simulink model "vsi_fmt_core"  (Simulink 7.0)
settings: Solver=ode45  StartTime=0.0  StopTime=10.0  RelTol=1e-3
libraries: xbsIndex_r4 x293, xbsReplacements_r4 x15, simulink x3, vlbi_lib x1
(part 2 of 2)

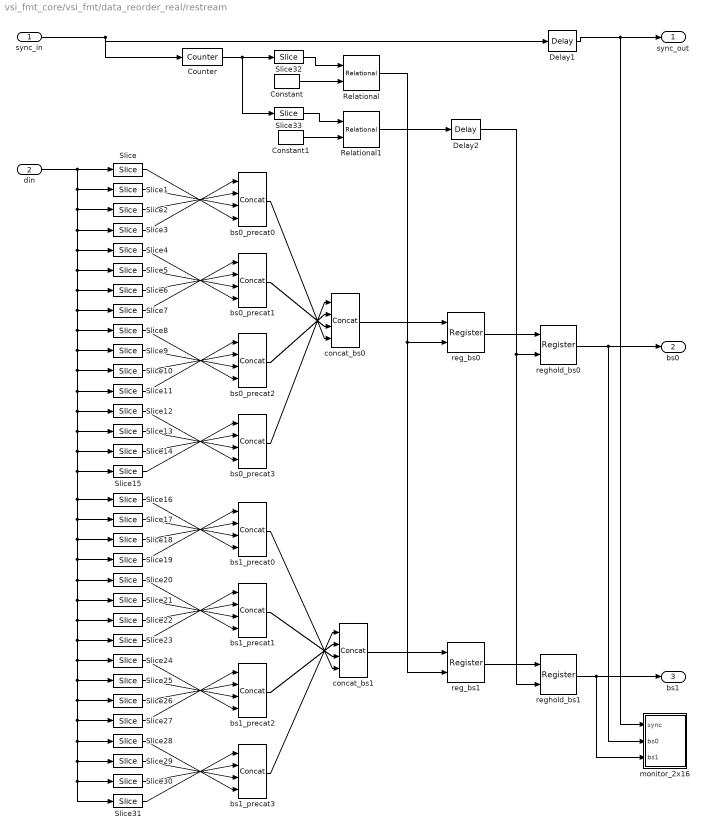
== system vsi_fmt_core/vsi_fmt/data_reorder_real/restream ==
  sync_in : Inport  OutDataType=sfix(16)  OutScaling=2^0
  din : Inport  Port=2  OutDataType=sfix(16)  OutScaling=2^0
  Constant : xbsIndex_r4/Constant  arith_type=Unsigned  const=0  n_bits=8-log2(clock_rate)  bin_pt=0  explicit_period=on  period=1  equ=P=C  opselect=C  inp2=PCIN>>17  opr=+  inp1=P  carry=CIN  dbl_ovrd=off  block_type=constant
      settings: block_version=11.3
  Constant1 : xbsIndex_r4/Constant  arith_type=Unsigned  const=0  n_bits=8-log2(clock_rate)  bin_pt=0  explicit_period=on  period=1  equ=P=C  opselect=C  inp2=PCIN>>17  opr=+  inp1=P  carry=CIN  dbl_ovrd=off  block_type=constant
      settings: block_version=11.3
  Counter : xbsIndex_r4/Counter  cnt_type=Free Running  cnt_to=Inf  operation=Up  start_count=0  cnt_by_val=1  arith_type=Unsigned  n_bits=9-log2(clock_rate)  bin_pt=0  load_pin=off  rst=on  en=off  explicit_period=off  period=1  dbl_ovrd=off  use_behavioral_HDL=off  use_rpm=on  implementation=Fabric  block_type=counter
      settings: xl_area=[0, 0, 0, 0, 0, 0, 0]  block_version=11.3
  Delay1 : xbsIndex_r4/Delay  en=off  latency=2  dbl_ovrd=off  reg_retiming=off  block_type=delay
      settings: xl_area=[0, 0, 0, 0, 0, 0, 0]  block_version=11.3
  Delay2 : xbsIndex_r4/Delay  en=off  latency=1  dbl_ovrd=off  reg_retiming=off  block_type=delay
      settings: xl_area=[0, 0, 0, 0, 0, 0, 0]  block_version=11.3
  Relational : xbsIndex_r4/Relational  mode=a=b  en=off  latency=0  dbl_ovrd=off  block_type=relational
      settings: xl_area=[0, 0, 0, 0, 0, 0, 0]  block_version=11.3
  Relational1 : xbsIndex_r4/Relational  mode=a=b  en=off  latency=0  dbl_ovrd=off  block_type=relational
      settings: xl_area=[0, 0, 0, 0, 0, 0, 0]  block_version=11.3
  Slice : xbsIndex_r4/Slice  nbits=sample_width  boolean_output=off  mode=Lower Bit Location + Width  bit1=sample_width*0  base1=MSB of Input  bit0=sample_width*7  base0=LSB of Input  dbl_ovrd=off  block_type=slice
      settings: block_version=11.3
  Slice1 : xbsIndex_r4/Slice  nbits=sample_width  boolean_output=off  mode=Lower Bit Location + Width  bit1=-2*sample_width  base1=MSB of Input  bit0=sample_width*6  base0=LSB of Input  dbl_ovrd=off  block_type=slice
      settings: block_version=11.3
  Slice10 : xbsIndex_r4/Slice  nbits=sample_width  boolean_output=off  mode=Lower Bit Location + Width  bit1=sample_width*21  base1=MSB of Input  bit0=sample_width*21  base0=LSB of Input  dbl_ovrd=off  block_type=slice
      settings: block_version=11.3
  Slice11 : xbsIndex_r4/Slice  nbits=sample_width  boolean_output=off  mode=Lower Bit Location + Width  bit1=-22*sample_width  base1=MSB of Input  bit0=sample_width*20  base0=LSB of Input  dbl_ovrd=off  block_type=slice
      settings: block_version=11.3
  Slice12 : xbsIndex_r4/Slice  nbits=sample_width  boolean_output=off  mode=Lower Bit Location + Width  bit1=-24*sample_width  base1=MSB of Input  bit0=sample_width*31  base0=LSB of Input  dbl_ovrd=off  block_type=slice
      settings: block_version=11.3
  Slice13 : xbsIndex_r4/Slice  nbits=sample_width  boolean_output=off  mode=Lower Bit Location + Width  bit1=-26*sample_width  base1=MSB of Input  bit0=sample_width*30  base0=LSB of Input  dbl_ovrd=off  block_type=slice
      settings: block_version=11.3
  Slice14 : xbsIndex_r4/Slice  nbits=sample_width  boolean_output=off  mode=Lower Bit Location + Width  bit1=-28*sample_width  base1=MSB of Input  bit0=sample_width*29  base0=LSB of Input  dbl_ovrd=off  block_type=slice
      settings: block_version=11.3
  Slice15 : xbsIndex_r4/Slice  nbits=sample_width  boolean_output=off  mode=Lower Bit Location + Width  bit1=-30*sample_width  base1=MSB of Input  bit0=sample_width*28  base0=LSB of Input  dbl_ovrd=off  block_type=slice
      settings: block_version=11.3
  Slice16 : xbsIndex_r4/Slice  nbits=sample_width  boolean_output=off  mode=Lower Bit Location + Width  bit1=-1*sample_width  base1=MSB of Input  bit0=sample_width*3  base0=LSB of Input  dbl_ovrd=off  block_type=slice
      settings: block_version=11.3
  Slice17 : xbsIndex_r4/Slice  nbits=sample_width  boolean_output=off  mode=Lower Bit Location + Width  bit1=-3*sample_width  base1=MSB of Input  bit0=sample_width*2  base0=LSB of Input  dbl_ovrd=off  block_type=slice
      settings: block_version=11.3
  Slice18 : xbsIndex_r4/Slice  nbits=sample_width  boolean_output=off  mode=Lower Bit Location + Width  bit1=-5*sample_width  base1=MSB of Input  bit0=sample_width*1  base0=LSB of Input  dbl_ovrd=off  block_type=slice
      settings: block_version=11.3
  Slice19 : xbsIndex_r4/Slice  nbits=sample_width  boolean_output=off  mode=Lower Bit Location + Width  bit1=-7*sample_width  base1=MSB of Input  bit0=sample_width*0  base0=LSB of Input  dbl_ovrd=off  block_type=slice
      settings: block_version=11.3
  Slice2 : xbsIndex_r4/Slice  nbits=sample_width  boolean_output=off  mode=Lower Bit Location + Width  bit1=-4*sample_width  base1=MSB of Input  bit0=sample_width*5  base0=LSB of Input  dbl_ovrd=off  block_type=slice
      settings: block_version=11.3
  Slice20 : xbsIndex_r4/Slice  nbits=sample_width  boolean_output=off  mode=Lower Bit Location + Width  bit1=-9*sample_width  base1=MSB of Input  bit0=sample_width*11  base0=LSB of Input  dbl_ovrd=off  block_type=slice
      settings: block_version=11.3
  Slice21 : xbsIndex_r4/Slice  nbits=sample_width  boolean_output=off  mode=Lower Bit Location + Width  bit1=-11*sample_width  base1=MSB of Input  bit0=sample_width*10  base0=LSB of Input  dbl_ovrd=off  block_type=slice
      settings: block_version=11.3
  Slice22 : xbsIndex_r4/Slice  nbits=sample_width  boolean_output=off  mode=Lower Bit Location + Width  bit1=-13*sample_width  base1=MSB of Input  bit0=sample_width*9  base0=LSB of Input  dbl_ovrd=off  block_type=slice
      settings: block_version=11.3
  Slice23 : xbsIndex_r4/Slice  nbits=sample_width  boolean_output=off  mode=Lower Bit Location + Width  bit1=-15*sample_width  base1=MSB of Input  bit0=sample_width*8  base0=LSB of Input  dbl_ovrd=off  block_type=slice
      settings: block_version=11.3
  Slice24 : xbsIndex_r4/Slice  nbits=sample_width  boolean_output=off  mode=Lower Bit Location + Width  bit1=-17*sample_width  base1=MSB of Input  bit0=sample_width*19  base0=LSB of Input  dbl_ovrd=off  block_type=slice
      settings: block_version=11.3
  Slice25 : xbsIndex_r4/Slice  nbits=sample_width  boolean_output=off  mode=Lower Bit Location + Width  bit1=sample_width*18  base1=MSB of Input  bit0=sample_width*18  base0=LSB of Input  dbl_ovrd=off  block_type=slice
      settings: block_version=11.3
  Slice26 : xbsIndex_r4/Slice  nbits=sample_width  boolean_output=off  mode=Lower Bit Location + Width  bit1=-21*sample_width  base1=MSB of Input  bit0=sample_width*17  base0=LSB of Input  dbl_ovrd=off  block_type=slice
      settings: block_version=11.3
  Slice27 : xbsIndex_r4/Slice  nbits=sample_width  boolean_output=off  mode=Lower Bit Location + Width  bit1=-23*sample_width  base1=MSB of Input  bit0=sample_width*16  base0=LSB of Input  dbl_ovrd=off  block_type=slice
      settings: block_version=11.3
  Slice28 : xbsIndex_r4/Slice  nbits=sample_width  boolean_output=off  mode=Lower Bit Location + Width  bit1=-25*sample_width  base1=MSB of Input  bit0=sample_width*27  base0=LSB of Input  dbl_ovrd=off  block_type=slice
      settings: block_version=11.3
  Slice29 : xbsIndex_r4/Slice  nbits=sample_width  boolean_output=off  mode=Lower Bit Location + Width  bit1=-27*sample_width  base1=MSB of Input  bit0=sample_width*26  base0=LSB of Input  dbl_ovrd=off  block_type=slice
      settings: block_version=11.3
  Slice3 : xbsIndex_r4/Slice  nbits=sample_width  boolean_output=off  mode=Lower Bit Location + Width  bit1=-6*sample_width  base1=MSB of Input  bit0=sample_width*4  base0=LSB of Input  dbl_ovrd=off  block_type=slice
      settings: block_version=11.3
  Slice30 : xbsIndex_r4/Slice  nbits=sample_width  boolean_output=off  mode=Lower Bit Location + Width  bit1=-29*sample_width  base1=MSB of Input  bit0=sample_width*25  base0=LSB of Input  dbl_ovrd=off  block_type=slice
      settings: block_version=11.3
  Slice31 : xbsIndex_r4/Slice  nbits=sample_width  boolean_output=off  mode=Lower Bit Location + Width  bit1=-31*sample_width  base1=MSB of Input  bit0=sample_width*24  base0=LSB of Input  dbl_ovrd=off  block_type=slice
      settings: block_version=11.3
  Slice32 : xbsIndex_r4/Slice  nbits=8-log2(clock_rate)  boolean_output=off  mode=Upper Bit Location + Width  bit1=0  base1=MSB of Input  bit0=sample_width*7  base0=LSB of Input  dbl_ovrd=off  block_type=slice
      settings: block_version=11.3
  Slice33 : xbsIndex_r4/Slice  nbits=8-log2(clock_rate)  boolean_output=off  mode=Lower Bit Location + Width  bit1=0  base1=MSB of Input  bit0=0  base0=LSB of Input  dbl_ovrd=off  block_type=slice
      settings: block_version=11.3
  Slice4 : xbsIndex_r4/Slice  nbits=sample_width  boolean_output=off  mode=Lower Bit Location + Width  bit1=-8*sample_width  base1=MSB of Input  bit0=sample_width*15  base0=LSB of Input  dbl_ovrd=off  block_type=slice
      settings: block_version=11.3
  Slice5 : xbsIndex_r4/Slice  nbits=sample_width  boolean_output=off  mode=Lower Bit Location + Width  bit1=-10*sample_width  base1=MSB of Input  bit0=sample_width*14  base0=LSB of Input  dbl_ovrd=off  block_type=slice
      settings: block_version=11.3
  Slice6 : xbsIndex_r4/Slice  nbits=sample_width  boolean_output=off  mode=Lower Bit Location + Width  bit1=-12*sample_width  base1=MSB of Input  bit0=sample_width*13  base0=LSB of Input  dbl_ovrd=off  block_type=slice
      settings: block_version=11.3
  Slice7 : xbsIndex_r4/Slice  nbits=sample_width  boolean_output=off  mode=Lower Bit Location + Width  bit1=-14*sample_width  base1=MSB of Input  bit0=sample_width*12  base0=LSB of Input  dbl_ovrd=off  block_type=slice
      settings: block_version=11.3
  Slice8 : xbsIndex_r4/Slice  nbits=sample_width  boolean_output=off  mode=Lower Bit Location + Width  bit1=-16*sample_width  base1=MSB of Input  bit0=sample_width*23  base0=LSB of Input  dbl_ovrd=off  block_type=slice
      settings: block_version=11.3
  Slice9 : xbsIndex_r4/Slice  nbits=sample_width  boolean_output=off  mode=Lower Bit Location + Width  bit1=-18*sample_width  base1=MSB of Input  bit0=sample_width*22  base0=LSB of Input  dbl_ovrd=off  block_type=slice
      settings: block_version=11.3
  bs0_precat{0..3} (4 alike) : xbsIndex_r4/Concat  num_inputs=4  dbl_ovrd=off  block_type=concat
      settings: block_version=11.3
  bs1_precat{0..3} (4 alike) : xbsIndex_r4/Concat  num_inputs=4  dbl_ovrd=off  block_type=concat
      settings: block_version=11.3
  concat_bs0 : xbsIndex_r4/Concat  num_inputs=4  dbl_ovrd=off  block_type=concat
      settings: block_version=11.3
  concat_bs1 : xbsIndex_r4/Concat  num_inputs=4  dbl_ovrd=off  block_type=concat
      settings: block_version=11.3
  monitor_2x16 : Subsystem
  reg_bs0 : xbsIndex_r4/Register  init=0  rst=off  en=on  dbl_ovrd=off  block_type=register
      settings: xl_area=[0, 0, 0, 0, 0, 0, 0]  block_version=11.3
  reg_bs1 : xbsIndex_r4/Register  init=0  rst=off  en=on  dbl_ovrd=off  block_type=register
      settings: xl_area=[0, 0, 0, 0, 0, 0, 0]  block_version=11.3
  reghold_bs0 : xbsIndex_r4/Register  init=0  rst=off  en=on  dbl_ovrd=off  block_type=register
      settings: xl_area=[0, 0, 0, 0, 0, 0, 0]  block_version=11.3
  reghold_bs1 : xbsIndex_r4/Register  init=0  rst=off  en=on  dbl_ovrd=off  block_type=register
      settings: xl_area=[0, 0, 0, 0, 0, 0, 0]  block_version=11.3
  sync_out : Outport  OutDataType=sfix(16)  OutScaling=2^0
  bs0 : Outport  Port=2  OutDataType=sfix(16)  OutScaling=2^0
  bs1 : Outport  Port=3  OutDataType=sfix(16)  OutScaling=2^0
  wires:
  Delay2/1 -> reghold_bs1/2, reghold_bs0/2
  Relational1/1 -> Delay2/1
  Slice33/1 -> Relational1/1
  Constant1/1 -> Relational1/2
  Slice32/1 -> Relational/1
  Counter/1 -> Slice33/1, Slice32/1
  reghold_bs1/1 -> monitor_2x16/3(bs1), bs1/1
  reghold_bs0/1 -> monitor_2x16/2(bs0), bs0/1
  Delay1/1 -> monitor_2x16/1(sync), sync_out/1
  reg_bs1/1 -> reghold_bs1/1
  reg_bs0/1 -> reghold_bs0/1
  Relational/1 -> reg_bs1/2, reg_bs0/2
  Constant/1 -> Relational/2
  sync_in/1 -> Delay1/1, Counter/1
  din/1 -> Slice6/1, Slice7/1, Slice14/1, Slice15/1, Slice16/1, Slice17/1, Slice18/1, Slice19/1, Slice20/1, Slice21/1, Slice24/1, Slice25/1, Slice26/1, Slice27/1, Slice28/1, Slice29/1, Slice30/1, Slice31/1, Slice23/1, Slice22/1, Slice13/1, Slice12/1, Slice11/1, Slice10/1, Slice9/1, Slice8/1, Slice5/1, Slice4/1, Slice3/1, Slice2/1, Slice1/1, Slice/1
  Slice/1 -> bs0_precat0/4
  Slice1/1 -> bs0_precat0/3
  Slice2/1 -> bs0_precat0/2
  Slice3/1 -> bs0_precat0/1
  Slice4/1 -> bs0_precat1/4
  Slice5/1 -> bs0_precat1/3
  Slice6/1 -> bs0_precat1/2
  Slice7/1 -> bs0_precat1/1
  Slice8/1 -> bs0_precat2/4
  Slice9/1 -> bs0_precat2/3
  Slice10/1 -> bs0_precat2/2
  Slice11/1 -> bs0_precat2/1
  Slice12/1 -> bs0_precat3/4
  Slice13/1 -> bs0_precat3/3
  Slice14/1 -> bs0_precat3/2
  Slice15/1 -> bs0_precat3/1
  Slice16/1 -> bs1_precat0/4
  Slice17/1 -> bs1_precat0/3
  Slice18/1 -> bs1_precat0/2
  Slice19/1 -> bs1_precat0/1
  Slice20/1 -> bs1_precat1/4
  Slice21/1 -> bs1_precat1/3
  Slice22/1 -> bs1_precat1/2
  Slice23/1 -> bs1_precat1/1
  Slice24/1 -> bs1_precat2/4
  Slice25/1 -> bs1_precat2/3
  Slice26/1 -> bs1_precat2/2
  Slice27/1 -> bs1_precat2/1
  Slice28/1 -> bs1_precat3/4
  Slice29/1 -> bs1_precat3/3
  Slice30/1 -> bs1_precat3/2
  Slice31/1 -> bs1_precat3/1
  concat_bs0/1 -> reg_bs0/1
  concat_bs1/1 -> reg_bs1/1
  bs0_precat0/1 -> concat_bs0/4
  bs0_precat1/1 -> concat_bs0/3
  bs0_precat2/1 -> concat_bs0/2
  bs0_precat3/1 -> concat_bs0/1
  bs1_precat0/1 -> concat_bs1/4
  bs1_precat1/1 -> concat_bs1/3
  bs1_precat2/1 -> concat_bs1/2
  bs1_precat3/1 -> concat_bs1/1

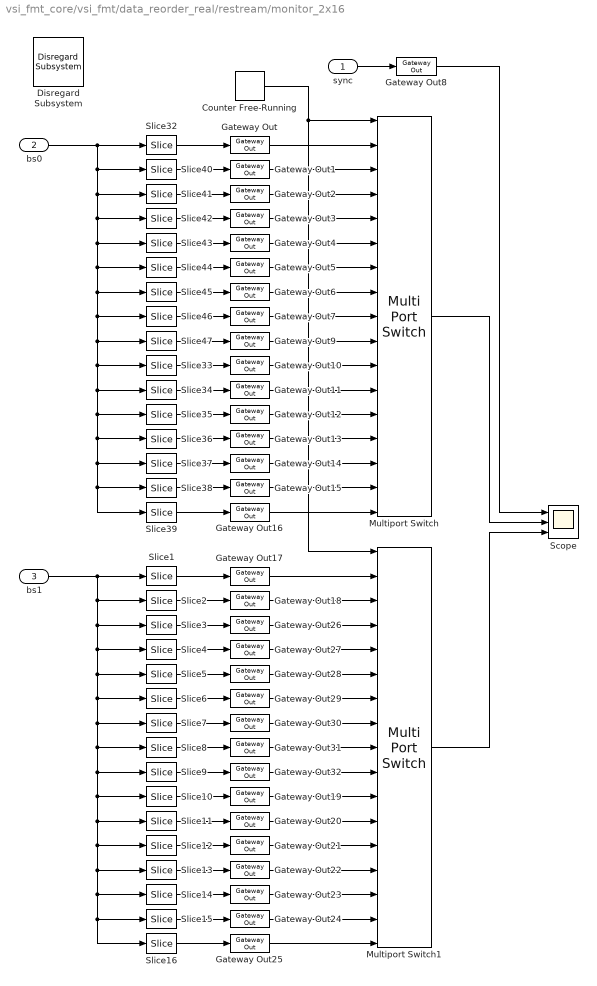
== system vsi_fmt_core/vsi_fmt/data_reorder_real/restream/monitor_2x16 ==
  sync : Inport  OutDataType=sfix(16)  OutScaling=2^0
  bs0 : Inport  Port=2  OutDataType=sfix(16)  OutScaling=2^0
  bs1 : Inport  Port=3  OutDataType=sfix(16)  OutScaling=2^0
  Counter Free-Running : simulink/Sources/Counter Free-Running  SystemSampleTime=-1  NumBits=4  tsamp=1/16
  Disregard Subsystem : xbsIndex_r4/Disregard Subsystem  Tag=discardX  block_type=disregard
      settings: block_version=11.3
  Gateway Out{,1..32} (33 alike) : xbsIndex_r4/Gateway Out  hdl_port=off  timing_constraint=None  locs_specified=off  LOCs={}  block_type=gatewayout
      settings: infoedit="Gateway out block.  Converts Xilinx fixed point inputs into ouputs of type Simulink integer, double, or fixed point.<br><br>Hardware notes:  In hardware these blocks become top level output ports or are discarded, depending on how they are configured."  xl_area=[0, 0, 0, 0, 0, 0, 0]  block_version=11.3
  Multiport Switch : MultiPortSwitch  Inputs=16  zeroidx=on  SampleTime=1/16
  Multiport Switch1 : MultiPortSwitch  Inputs=16  zeroidx=on  SampleTime=1/16
  Scope : Scope  NumInputPorts=3
      settings: YMin=-5~-5~-5  YMax=5~5~5
  Slice1 : xbsIndex_r4/Slice  nbits=sample_width  boolean_output=off  mode=Upper Bit Location + Width  bit1=sample_width * 0  base1=MSB of Input  bit0=0  base0=LSB of Input  dbl_ovrd=off  block_type=slice
      settings: block_version=11.3
  Slice10 : xbsIndex_r4/Slice  nbits=sample_width  boolean_output=off  mode=Upper Bit Location + Width  bit1=sample_width * -9  base1=MSB of Input  bit0=0  base0=LSB of Input  dbl_ovrd=off  block_type=slice
      settings: block_version=11.3
  Slice11 : xbsIndex_r4/Slice  nbits=sample_width  boolean_output=off  mode=Upper Bit Location + Width  bit1=sample_width * -10  base1=MSB of Input  bit0=0  base0=LSB of Input  dbl_ovrd=off  block_type=slice
      settings: block_version=11.3
  Slice12 : xbsIndex_r4/Slice  nbits=sample_width  boolean_output=off  mode=Upper Bit Location + Width  bit1=sample_width * -11  base1=MSB of Input  bit0=0  base0=LSB of Input  dbl_ovrd=off  block_type=slice
      settings: block_version=11.3
  Slice13 : xbsIndex_r4/Slice  nbits=sample_width  boolean_output=off  mode=Upper Bit Location + Width  bit1=sample_width * -12  base1=MSB of Input  bit0=0  base0=LSB of Input  dbl_ovrd=off  block_type=slice
      settings: block_version=11.3
  Slice14 : xbsIndex_r4/Slice  nbits=sample_width  boolean_output=off  mode=Upper Bit Location + Width  bit1=sample_width * -13  base1=MSB of Input  bit0=0  base0=LSB of Input  dbl_ovrd=off  block_type=slice
      settings: block_version=11.3
  Slice15 : xbsIndex_r4/Slice  nbits=sample_width  boolean_output=off  mode=Upper Bit Location + Width  bit1=sample_width * -14  base1=MSB of Input  bit0=0  base0=LSB of Input  dbl_ovrd=off  block_type=slice
      settings: block_version=11.3
  Slice16 : xbsIndex_r4/Slice  nbits=sample_width  boolean_output=off  mode=Upper Bit Location + Width  bit1=sample_width * -15  base1=MSB of Input  bit0=0  base0=LSB of Input  dbl_ovrd=off  block_type=slice
      settings: block_version=11.3
  Slice2 : xbsIndex_r4/Slice  nbits=sample_width  boolean_output=off  mode=Upper Bit Location + Width  bit1=sample_width * -1  base1=MSB of Input  bit0=0  base0=LSB of Input  dbl_ovrd=off  block_type=slice
      settings: block_version=11.3
  Slice3 : xbsIndex_r4/Slice  nbits=sample_width  boolean_output=off  mode=Upper Bit Location + Width  bit1=sample_width * -2  base1=MSB of Input  bit0=0  base0=LSB of Input  dbl_ovrd=off  block_type=slice
      settings: block_version=11.3
  Slice32 : xbsIndex_r4/Slice  nbits=sample_width  boolean_output=off  mode=Upper Bit Location + Width  bit1=sample_width * 0  base1=MSB of Input  bit0=0  base0=LSB of Input  dbl_ovrd=off  block_type=slice
      settings: block_version=11.3
  Slice33 : xbsIndex_r4/Slice  nbits=sample_width  boolean_output=off  mode=Upper Bit Location + Width  bit1=sample_width * -9  base1=MSB of Input  bit0=0  base0=LSB of Input  dbl_ovrd=off  block_type=slice
      settings: block_version=11.3
  Slice34 : xbsIndex_r4/Slice  nbits=sample_width  boolean_output=off  mode=Upper Bit Location + Width  bit1=sample_width * -10  base1=MSB of Input  bit0=0  base0=LSB of Input  dbl_ovrd=off  block_type=slice
      settings: block_version=11.3
  Slice35 : xbsIndex_r4/Slice  nbits=sample_width  boolean_output=off  mode=Upper Bit Location + Width  bit1=sample_width * -11  base1=MSB of Input  bit0=0  base0=LSB of Input  dbl_ovrd=off  block_type=slice
      settings: block_version=11.3
  Slice36 : xbsIndex_r4/Slice  nbits=sample_width  boolean_output=off  mode=Upper Bit Location + Width  bit1=sample_width * -12  base1=MSB of Input  bit0=0  base0=LSB of Input  dbl_ovrd=off  block_type=slice
      settings: block_version=11.3
  Slice37 : xbsIndex_r4/Slice  nbits=sample_width  boolean_output=off  mode=Upper Bit Location + Width  bit1=sample_width * -13  base1=MSB of Input  bit0=0  base0=LSB of Input  dbl_ovrd=off  block_type=slice
      settings: block_version=11.3
  Slice38 : xbsIndex_r4/Slice  nbits=sample_width  boolean_output=off  mode=Upper Bit Location + Width  bit1=sample_width * -14  base1=MSB of Input  bit0=0  base0=LSB of Input  dbl_ovrd=off  block_type=slice
      settings: block_version=11.3
  Slice39 : xbsIndex_r4/Slice  nbits=sample_width  boolean_output=off  mode=Upper Bit Location + Width  bit1=sample_width * -15  base1=MSB of Input  bit0=0  base0=LSB of Input  dbl_ovrd=off  block_type=slice
      settings: block_version=11.3
  Slice4 : xbsIndex_r4/Slice  nbits=sample_width  boolean_output=off  mode=Upper Bit Location + Width  bit1=sample_width * -3  base1=MSB of Input  bit0=0  base0=LSB of Input  dbl_ovrd=off  block_type=slice
      settings: block_version=11.3
  Slice40 : xbsIndex_r4/Slice  nbits=sample_width  boolean_output=off  mode=Upper Bit Location + Width  bit1=sample_width * -1  base1=MSB of Input  bit0=0  base0=LSB of Input  dbl_ovrd=off  block_type=slice
      settings: block_version=11.3
  Slice41 : xbsIndex_r4/Slice  nbits=sample_width  boolean_output=off  mode=Upper Bit Location + Width  bit1=sample_width * -2  base1=MSB of Input  bit0=0  base0=LSB of Input  dbl_ovrd=off  block_type=slice
      settings: block_version=11.3
  Slice42 : xbsIndex_r4/Slice  nbits=sample_width  boolean_output=off  mode=Upper Bit Location + Width  bit1=sample_width * -3  base1=MSB of Input  bit0=0  base0=LSB of Input  dbl_ovrd=off  block_type=slice
      settings: block_version=11.3
  Slice43 : xbsIndex_r4/Slice  nbits=sample_width  boolean_output=off  mode=Upper Bit Location + Width  bit1=sample_width * -4  base1=MSB of Input  bit0=0  base0=LSB of Input  dbl_ovrd=off  block_type=slice
      settings: block_version=11.3
  Slice44 : xbsIndex_r4/Slice  nbits=sample_width  boolean_output=off  mode=Upper Bit Location + Width  bit1=sample_width * -5  base1=MSB of Input  bit0=0  base0=LSB of Input  dbl_ovrd=off  block_type=slice
      settings: block_version=11.3
  Slice45 : xbsIndex_r4/Slice  nbits=sample_width  boolean_output=off  mode=Upper Bit Location + Width  bit1=sample_width * -6  base1=MSB of Input  bit0=0  base0=LSB of Input  dbl_ovrd=off  block_type=slice
      settings: block_version=11.3
  Slice46 : xbsIndex_r4/Slice  nbits=sample_width  boolean_output=off  mode=Upper Bit Location + Width  bit1=sample_width * -7  base1=MSB of Input  bit0=0  base0=LSB of Input  dbl_ovrd=off  block_type=slice
      settings: block_version=11.3
  Slice47 : xbsIndex_r4/Slice  nbits=sample_width  boolean_output=off  mode=Upper Bit Location + Width  bit1=sample_width * -8  base1=MSB of Input  bit0=0  base0=LSB of Input  dbl_ovrd=off  block_type=slice
      settings: block_version=11.3
  Slice5 : xbsIndex_r4/Slice  nbits=sample_width  boolean_output=off  mode=Upper Bit Location + Width  bit1=sample_width * -4  base1=MSB of Input  bit0=0  base0=LSB of Input  dbl_ovrd=off  block_type=slice
      settings: block_version=11.3
  Slice6 : xbsIndex_r4/Slice  nbits=sample_width  boolean_output=off  mode=Upper Bit Location + Width  bit1=sample_width * -5  base1=MSB of Input  bit0=0  base0=LSB of Input  dbl_ovrd=off  block_type=slice
      settings: block_version=11.3
  Slice7 : xbsIndex_r4/Slice  nbits=sample_width  boolean_output=off  mode=Upper Bit Location + Width  bit1=sample_width * -6  base1=MSB of Input  bit0=0  base0=LSB of Input  dbl_ovrd=off  block_type=slice
      settings: block_version=11.3
  Slice8 : xbsIndex_r4/Slice  nbits=sample_width  boolean_output=off  mode=Upper Bit Location + Width  bit1=sample_width * -7  base1=MSB of Input  bit0=0  base0=LSB of Input  dbl_ovrd=off  block_type=slice
      settings: block_version=11.3
  Slice9 : xbsIndex_r4/Slice  nbits=sample_width  boolean_output=off  mode=Upper Bit Location + Width  bit1=sample_width * -8  base1=MSB of Input  bit0=0  base0=LSB of Input  dbl_ovrd=off  block_type=slice
      settings: block_version=11.3
  wires:
  bs1/1 -> Slice16/1, Slice15/1, Slice14/1, Slice13/1, Slice12/1, Slice11/1, Slice10/1, Slice9/1, Slice8/1, Slice7/1, Slice6/1, Slice5/1, Slice4/1, Slice3/1, Slice2/1, Slice1/1
  Multiport Switch1/1 -> Scope/3
  Multiport Switch/1 -> Scope/2
  Gateway Out8/1 -> Scope/1
  sync/1 -> Gateway Out8/1
  Gateway Out25/1 -> Multiport Switch1/17
  Gateway Out24/1 -> Multiport Switch1/16
  Gateway Out23/1 -> Multiport Switch1/15
  Gateway Out22/1 -> Multiport Switch1/14
  Gateway Out21/1 -> Multiport Switch1/13
  Gateway Out20/1 -> Multiport Switch1/12
  Gateway Out19/1 -> Multiport Switch1/11
  Gateway Out32/1 -> Multiport Switch1/10
  Gateway Out31/1 -> Multiport Switch1/9
  Gateway Out30/1 -> Multiport Switch1/8
  Gateway Out29/1 -> Multiport Switch1/7
  Gateway Out28/1 -> Multiport Switch1/6
  Gateway Out27/1 -> Multiport Switch1/5
  Gateway Out26/1 -> Multiport Switch1/4
  Gateway Out18/1 -> Multiport Switch1/3
  Gateway Out17/1 -> Multiport Switch1/2
  Gateway Out16/1 -> Multiport Switch/17
  Gateway Out15/1 -> Multiport Switch/16
  Gateway Out14/1 -> Multiport Switch/15
  Gateway Out13/1 -> Multiport Switch/14
  Gateway Out12/1 -> Multiport Switch/13
  Gateway Out11/1 -> Multiport Switch/12
  Gateway Out10/1 -> Multiport Switch/11
  Gateway Out9/1 -> Multiport Switch/10
  Gateway Out7/1 -> Multiport Switch/9
  Gateway Out6/1 -> Multiport Switch/8
  Gateway Out5/1 -> Multiport Switch/7
  Gateway Out4/1 -> Multiport Switch/6
  Gateway Out3/1 -> Multiport Switch/5
  Gateway Out2/1 -> Multiport Switch/4
  Gateway Out1/1 -> Multiport Switch/3
  Gateway Out/1 -> Multiport Switch/2
  Slice9/1 -> Gateway Out32/1
  Slice10/1 -> Gateway Out19/1
  Slice11/1 -> Gateway Out20/1
  Slice12/1 -> Gateway Out21/1
  Slice13/1 -> Gateway Out22/1
  Slice14/1 -> Gateway Out23/1
  Slice15/1 -> Gateway Out24/1
  Slice16/1 -> Gateway Out25/1
  Slice1/1 -> Gateway Out17/1
  Slice2/1 -> Gateway Out18/1
  Slice3/1 -> Gateway Out26/1
  Slice4/1 -> Gateway Out27/1
  Slice5/1 -> Gateway Out28/1
  Slice6/1 -> Gateway Out29/1
  Slice7/1 -> Gateway Out30/1
  Slice8/1 -> Gateway Out31/1
  Slice47/1 -> Gateway Out9/1
  Slice33/1 -> Gateway Out10/1
  Slice34/1 -> Gateway Out11/1
  Slice35/1 -> Gateway Out12/1
  Slice36/1 -> Gateway Out13/1
  Slice37/1 -> Gateway Out14/1
  Slice38/1 -> Gateway Out15/1
  Slice39/1 -> Gateway Out16/1
  bs0/1 -> Slice32/1, Slice40/1, Slice41/1, Slice42/1, Slice43/1, Slice44/1, Slice45/1, Slice46/1, Slice47/1, Slice33/1, Slice34/1, Slice35/1, Slice36/1, Slice37/1, Slice39/1, Slice38/1
  Slice32/1 -> Gateway Out/1
  Slice40/1 -> Gateway Out1/1
  Slice41/1 -> Gateway Out2/1
  Slice42/1 -> Gateway Out3/1
  Slice43/1 -> Gateway Out4/1
  Slice44/1 -> Gateway Out5/1
  Slice45/1 -> Gateway Out6/1
  Slice46/1 -> Gateway Out7/1
  Counter Free-Running/1 -> Multiport Switch1/1, Multiport Switch/1
